simulink model "project2Linear"  (R2018b)
settings: Solver=VariableStepAuto  StartTime=0.0  StopTime=7  RelTol=1e-3
settings Model: Creator=Young Wang  LastModifiedBy=Young Wang

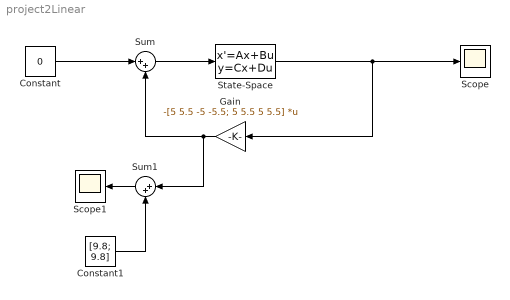
== system project2Linear ==
  Constant : Constant  Value=0
  Constant1 : Constant  Value=[9.8; 9.8]  VectorParams1D=off
  Gain : Gain  Gain=-[5 5.5 -5 -5.5; 5 5.5 5 5.5]  Multiplication=Matrix(K*u)
  Scope : Scope
  Scope1 : Scope
  State-Space : StateSpace  A=[0 1 0 0; 0 0 0 0; 0 0 0 1; 0 0 0 0]  B=[0 0; 1 1; 0 0; -1 1]  C=eye(4)  D=zeros(4,2)  InitialCondition=[1; 1; 1; 1]
  Sum : Sum  Inputs=|++
  Sum1 : Sum  Inputs=|++
  wires:
  Constant/1 -> Sum/1
  Gain/1 -> Sum1/1, Sum/2
  Sum/1 -> State-Space/1
  State-Space/1 -> Gain/1, Scope/1
  Constant1/1 -> Sum1/2
  Sum1/1 -> Scope1/1
